simulink model "PFC_Mathematicalmodel_MCHV3"  (R2022a)
settings: Solver=ode8  StartTime=0.0  StopTime=10  RelTol=1e-3
values from neighbouring files (symbols this model uses):
  C = 3*470e-6    (= 0.00141)    [PFC_Mathematicalmodel_MCHV3_data.m]
  Ki_i = Kp_i*2*pi*fz_i    (= 14162.3628627)    [PFC_Mathematicalmodel_MCHV3_data.m]
  Ki_v = Kp_v*2*pi*fz_v    (= 22.7249846961)    [PFC_Mathematicalmodel_MCHV3_data.m]
  KiL = 1/Ibase    (= 0.0469483568075)    [PFC_Mathematicalmodel_MCHV3_data.m]
  Kmul = Vpk_min/(2*Vbase)    (= 0.218498896247)    [PFC_Mathematicalmodel_MCHV3_data.m]
  Kp_i = Gci    (= 2.81751256932)    [PFC_Mathematicalmodel_MCHV3_data.m]
  Kp_v = Gcv    (= 3.61679364607)    [PFC_Mathematicalmodel_MCHV3_data.m]
  Kvin = 1/Vbase    (= 0.00220750551876)    [PFC_Mathematicalmodel_MCHV3_data.m]
  Kvo = 1/Vbase    (= 0.00220750551876)    [PFC_Mathematicalmodel_MCHV3_data.m]
  L = 1e-3    (= 0.001)    [PFC_Mathematicalmodel_MCHV3_data.m]
  R = (Vout^2)/Po    (= 144.4)    [PFC_Mathematicalmodel_MCHV3_data.m]
  Slope = (Vref-Vout_init)/T_rise    (= 273.9)    [PFC_Mathematicalmodel_MCHV3_data.m]
  Tsi = Isr / fsw    (= 1.25e-05)    [PFC_Mathematicalmodel_MCHV3_data.m]
  Tsv = Osr / fsw    (= 0.0002)    [PFC_Mathematicalmodel_MCHV3_data.m]
  Vin_pk = Vin_rms*1.414    (= 325.22)    [PFC_Mathematicalmodel_MCHV3_data.m]
  Vin_rms = 230    [PFC_Mathematicalmodel_MCHV3_data.m]
libraries: slpidlib x2, simulink x2, spsPWMGeneratorDCDCLib x1, spsRMSLib x1, spsMeanLib x1
settings Model: Creator=I50990  LastModifiedBy=I50990

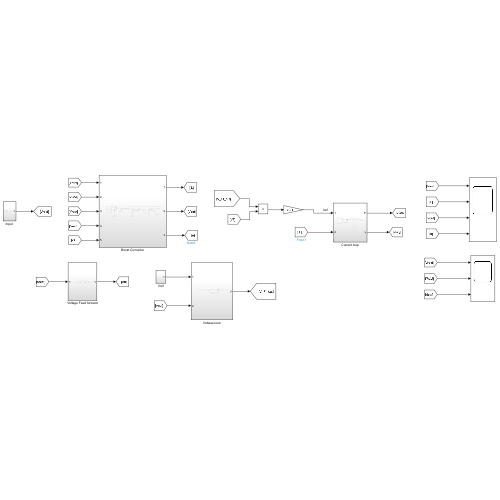
[thumbnail: Simulink's stored preview of the top-level diagram]
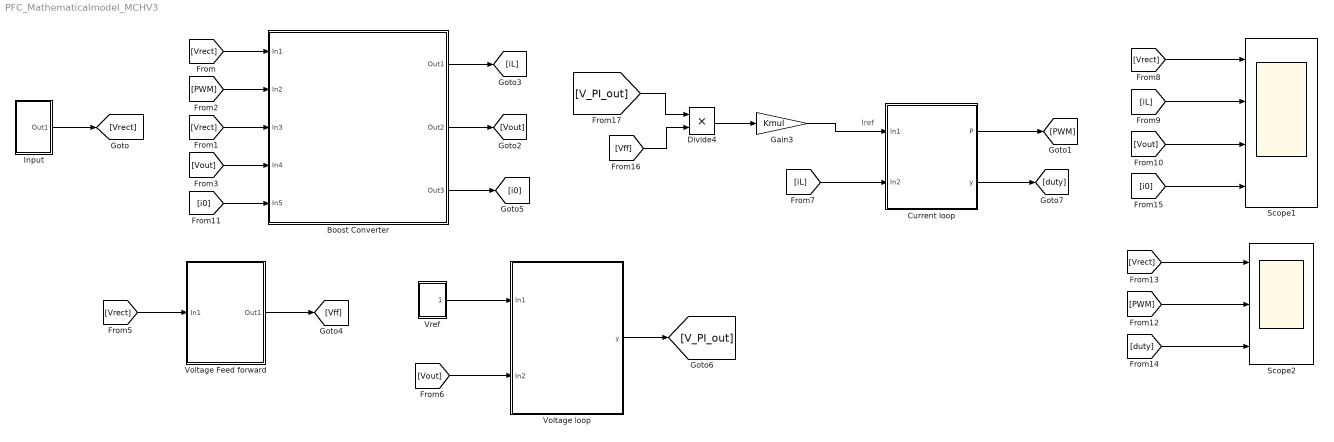
== system PFC_Mathematicalmodel_MCHV3 ==
  note: Iref
  Boost Converter : Subsystem
  Current loop : Subsystem
  Divide4 : Product  Inputs=**
  Gain3 : Gain  Gain=Kmul
  "Input " : Subsystem
  Scope1 : Scope  NumInputPorts=4
  Scope2 : Scope  NumInputPorts=3
  Voltage Feed forward : Subsystem
  Voltage loop : Subsystem
  Vref : Subsystem
  wires:
  Divide4/1 -> Gain3/1
  [Vrect] -> Scope1/1
  [iL] -> Scope1/2
  [Vout] -> Scope1/3
  [duty] -> Scope2/3
  [PWM] -> Scope2/2
  [Vrect] -> Scope2/1
  [i0] -> Scope1/4
  "Input "/1(Out1) -> [Vrect]
  [Vff] -> Divide4/2
  [V_PI_out] -> Divide4/1
  Vref/1(Out1) -> Voltage loop/1(In1)
  [Vout] -> Voltage loop/2(In2)
  Voltage loop/1(y) -> [V_PI_out]
  [Vrect] -> Boost Converter/1(In1)
  [PWM] -> Boost Converter/2(In2)
  [Vrect] -> Boost Converter/3(In3)
  [Vout] -> Boost Converter/4(In4)
  [i0] -> Boost Converter/5(In5)
  Boost Converter/1(Out1) -> [iL]
  Boost Converter/2(Out2) -> [Vout]
  Boost Converter/3(Out3) -> [i0]
  [Vrect] -> Voltage Feed forward/1(In1)
  Voltage Feed forward/1(Out1) -> [Vff]
  Gain3/1 -> Current loop/1(In1)
  [iL] -> Current loop/2(In2)
  Current loop/1(P) -> [PWM]
  Current loop/2(y) -> [duty]

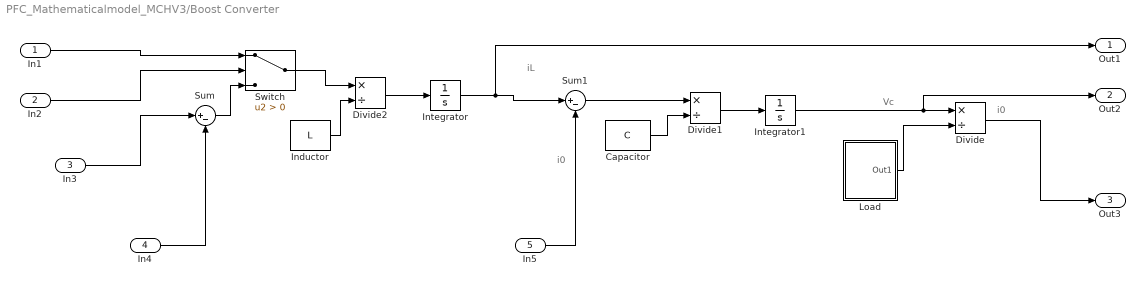
== system PFC_Mathematicalmodel_MCHV3/Boost Converter ==
  note: i0
  note: Vc
  note: i0
  note: iL
  In1 : Inport
  In2 : Inport  Port=2
  In3 : Inport  Port=3
  In4 : Inport  Port=4
  In5 : Inport  Port=5
  Capacitor : Constant  Value=C  SampleTime=Tsi
  Divide : Product  Inputs=*/
  Divide1 : Product  Inputs=*/
  Divide2 : Product  Inputs=*/
  Inductor : Constant  Value=L  SampleTime=Tsi
  Integrator : Integrator
  Integrator1 : Integrator  InitialCondition=Vin_pk
  Load : Subsystem
  Sum : Sum  Inputs=|+-
  Sum1 : Sum  Inputs=|+-
  Switch : Switch  Criteria=u2 > Threshold  SaturateOnIntegerOverflow=off  InputSameDT=off
  Out1 : Outport
  Out2 : Outport  Port=2
  Out3 : Outport  Port=3
  wires:
  Sum/1 -> Switch/3
  Integrator/1 -> Out1/1, Sum1/1
  In3/1 -> Sum/1
  Divide/1 -> Out3/1
  Integrator1/1 -> Out2/1, Divide/1
  Capacitor/1 -> Divide1/2
  In1/1 -> Switch/1
  Load/1(Out1) -> Divide/2
  Divide2/1 -> Integrator/1
  Divide1/1 -> Integrator1/1
  Switch/1 -> Divide2/1
  Sum1/1 -> Divide1/1
  Inductor/1 -> Divide2/2
  In5/1 -> Sum1/2
  In2/1 -> Switch/2
  In4/1 -> Sum/2

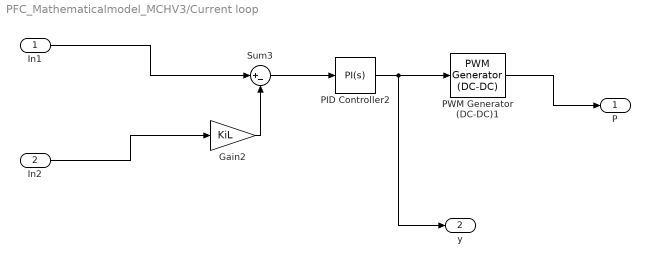
== system PFC_Mathematicalmodel_MCHV3/Current loop ==
  In1 : Inport
  In2 : Inport  Port=2
  Gain2 : Gain  Gain=KiL
  PID Controller2 : slpidlib/PID Controller  Controller=PI  Form=Parallel  TimeDomain=Continuous-time  UseExternalTs=off  SampleTime=-1  IntegratorMethod=Forward Euler  FilterMethod=Forward Euler  ControllerParametersSource=internal  P=Kp_i  I=Ki_i  UseKiTs=off  D=0  N=100  UseFilter=on  TunerSelectOption=Transfer Function Based (PID Tuner App)  ZeroCross=off  InitialConditionSource=internal  InitialConditionForIntegrator=0  InitialConditionForFilter=0  DifferentiatorICPrevScaledInput=0  ExternalReset=none  TrackingMode=off  Kt=1  LimitOutput=on  SatLimitsSource=internal  UpperSaturationLimit=0.95  LowerSaturationLimit=0  LinearizeAsGain=on  AntiWindupMode=none  Kb=1  POutMin=[]  POutMax=[]  IOutMin=[]  IOutMax=[]  DOutMin=[]  DOutMax=[]  NOutMin=[]  NOutMax=[]  SumOutMin=[]  SumOutMax=[]  SaturationOutMin=[]  SaturationOutMax=[]  PParamMin=[]  PParamMax=[]  IParamMin=[]  IParamMax=[]  DParamMin=[]  DParamMax=[]  NParamMin=[]  NParamMax=[]  KbParamMin=[]  KbParamMax=[]  KtParamMin=[]  KtParamMax=[]  KbOutMin=[]  KbOutMax=[]  KtOutMin=[]  KtOutMax=[]  IntegratorOutMin=[]  IntegratorOutMax=[]  FilterOutMin=[]  FilterOutMax=[]  SumI1OutMin=[]  SumI1OutMax=[]  SumI2OutMin=[]  SumI2OutMax=[]  SumI3OutMin=[]  SumI3OutMax=[]  SumI4OutMin=[]  SumI4OutMax=[]  SumDOutMin=[]  SumDOutMax=[]  DifferentiatorOutMin=[]  DifferentiatorOutMax=[]  FilterDiffOutCoefMin=[]  FilterDiffOutCoefMax=[]  ReciprocalOutMin=[]  ReciprocalOutMax=[]  SumDenOutMin=[]  SumDenOutMax=[]  SumNumOutMin=[]  SumNumOutMax=[]  DivideOutMin=[]  DivideOutMax=[]  UdiffTsProdOutMin=[]  UdiffTsProdOutMax=[]  NTsProdOutMin=[]  NTsProdOutMax=[]  UintegralTsProdOutMin=[]  UintegralTsProdOutMax=[]  UngainTsProdOutMin=[]  UngainTsProdOutMax=[]  IntegratorContinuousStateAttributes=''  IntegratorStateMustResolveToSignalObject=off  IntegratorRTWStateStorageClass=Auto  FilterContinuousStateAttributes=''  FilterStateMustResolveToSignalObject=off  FilterRTWStateStorageClass=Auto  ParallelPVariant=InternalParameters  IdealPVariant=Disabled  IVariant=InternalParameters  DVariant=Disabled  IntegratorVariant=Continuous  SatVariant=Enabled  AWVariant=Passthrough  PCopyVariant=Disabled  TRVariant=Disabled  FdbkBlocksVariant=Forward  IdealPFdbkVariant=Disabled  SatFdbkVariant=Disabled  DerivativeFilterVariant=Disabled  NVariant=Disabled  NCopyVariant=Disabled_SignalSpec  FilterICVariant=Disabled  IntegratorICVariant=InternalICs  ExternalResetVariant=Disabled  TRSumVariant=Passthrough  SumFdbkVariant=Disabled  SumVariant=Sum_PI  TsampFilterVariant=InternalTs  TsampNgainVariant=Passthrough  TsampIntegralVariant=Passthrough  ExternalSaturationOutDataTypeStr=Inherit: Same as second input  aMode=0
  PWM Generator (DC-DC)1 : spsPWMGeneratorDCDCLib/PWM Generator (DC-DC)  Fsw=fsw  Ts=Tsi/10
  Sum3 : Sum  Inputs=|+-
  P : Outport
  y : Outport  Port=2
  wires:
  Gain2/1 -> Sum3/2
  In2/1 -> Gain2/1
  Sum3/1 -> PID Controller2/1
  In1/1 -> Sum3/1
  PID Controller2/1 -> y/1, PWM Generator (DC-DC)1/1
  PWM Generator (DC-DC)1/1 -> P/1

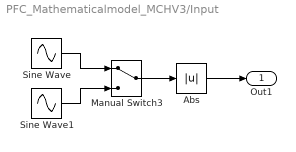
== system PFC_Mathematicalmodel_MCHV3/Input  ==
  Abs : Abs  SaturateOnIntegerOverflow=off
  Manual Switch3 : ManualSwitch
  Sine Wave : Sin  Amplitude=Vin_pk  Frequency=2*pi*50  SampleTime=0
  Sine Wave1 : Sin  Amplitude=Vin_pk/2  Frequency=2*pi*50  SampleTime=0
  Out1 : Outport
  wires:
  Sine Wave/1 -> Manual Switch3/1
  Manual Switch3/1 -> Abs/1
  Sine Wave1/1 -> Manual Switch3/2
  Abs/1 -> Out1/1

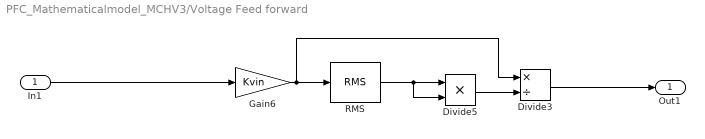
== system PFC_Mathematicalmodel_MCHV3/Voltage Feed forward ==
  In1 : Inport
  Divide3 : Product  Inputs=*/
  Divide5 : Product  Inputs=**
  Gain6 : Gain  Gain=Kvin
  RMS : spsRMSLib/RMS  TrueRMS=on  Freq=100  RMSInit=Vin_rms*Kvin  Ts=Tsi
  Out1 : Outport
  wires:
  RMS/1 -> Divide5/2, Divide5/1
  Gain6/1 -> Divide3/1, RMS/1
  Divide3/1 -> Out1/1
  Divide5/1 -> Divide3/2
  In1/1 -> Gain6/1

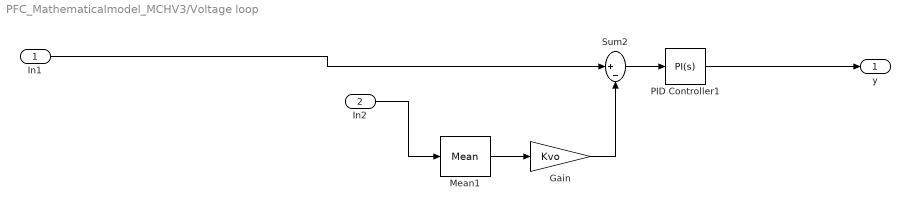
== system PFC_Mathematicalmodel_MCHV3/Voltage loop ==
  In1 : Inport
  In2 : Inport  Port=2
  Gain : Gain  Gain=Kvo
  Mean1 : spsMeanLib/Mean  Freq=100  Vinit=Vin_pk  Ts=Tsv
  PID Controller1 : slpidlib/PID Controller  Controller=PI  Form=Parallel  TimeDomain=Continuous-time  UseExternalTs=off  SampleTime=-1  IntegratorMethod=Forward Euler  FilterMethod=Forward Euler  ControllerParametersSource=internal  P=Kp_v  I=Ki_v  UseKiTs=off  D=0  N=100  UseFilter=on  TunerSelectOption=Transfer Function Based (PID Tuner App)  InitialConditionSource=internal  InitialConditionForIntegrator=0  InitialConditionForFilter=0  DifferentiatorICPrevScaledInput=0  ExternalReset=none  TrackingMode=off  Kt=1  LimitOutput=on  SatLimitsSource=internal  UpperSaturationLimit=1  LowerSaturationLimit=0  LinearizeAsGain=on  AntiWindupMode=none  Kb=1  POutMin=[]  POutMax=[]  IOutMin=[]  IOutMax=[]  DOutMin=[]  DOutMax=[]  NOutMin=[]  NOutMax=[]  SumOutMin=[]  SumOutMax=[]  SaturationOutMin=[]  SaturationOutMax=[]  PParamMin=[]  PParamMax=[]  IParamMin=[]  IParamMax=[]  DParamMin=[]  DParamMax=[]  NParamMin=[]  NParamMax=[]  KbParamMin=[]  KbParamMax=[]  KtParamMin=[]  KtParamMax=[]  KbOutMin=[]  KbOutMax=[]  KtOutMin=[]  KtOutMax=[]  IntegratorOutMin=[]  IntegratorOutMax=[]  FilterOutMin=[]  FilterOutMax=[]  SumI1OutMin=[]  SumI1OutMax=[]  SumI2OutMin=[]  SumI2OutMax=[]  SumI3OutMin=[]  SumI3OutMax=[]  SumI4OutMin=[]  SumI4OutMax=[]  SumDOutMin=[]  SumDOutMax=[]  DifferentiatorOutMin=[]  DifferentiatorOutMax=[]  FilterDiffOutCoefMin=[]  FilterDiffOutCoefMax=[]  ReciprocalOutMin=[]  ReciprocalOutMax=[]  SumDenOutMin=[]  SumDenOutMax=[]  SumNumOutMin=[]  SumNumOutMax=[]  DivideOutMin=[]  DivideOutMax=[]  UdiffTsProdOutMin=[]  UdiffTsProdOutMax=[]  NTsProdOutMin=[]  NTsProdOutMax=[]  UintegralTsProdOutMin=[]  UintegralTsProdOutMax=[]  UngainTsProdOutMin=[]  UngainTsProdOutMax=[]  IntegratorContinuousStateAttributes=''  IntegratorStateMustResolveToSignalObject=off  IntegratorRTWStateStorageClass=Auto  FilterContinuousStateAttributes=''  FilterStateMustResolveToSignalObject=off  FilterRTWStateStorageClass=Auto  ParallelPVariant=InternalParameters  IdealPVariant=Disabled  IVariant=InternalParameters  DVariant=Disabled  IntegratorVariant=Continuous  SatVariant=Enabled  AWVariant=Passthrough  PCopyVariant=Disabled  TRVariant=Disabled  FdbkBlocksVariant=Forward  IdealPFdbkVariant=Disabled  SatFdbkVariant=Disabled  DerivativeFilterVariant=Disabled  NVariant=Disabled  NCopyVariant=Disabled_SignalSpec  FilterICVariant=Disabled  IntegratorICVariant=InternalICs  ExternalResetVariant=Disabled  TRSumVariant=Passthrough  SumFdbkVariant=Disabled  SumVariant=Sum_PI  TsampFilterVariant=InternalTs  TsampNgainVariant=Passthrough  TsampIntegralVariant=Passthrough  ExternalSaturationOutDataTypeStr=Inherit: Same as second input  aMode=0
  Sum2 : Sum  Inputs=|+-
  y : Outport
  wires:
  In2/1 -> Mean1/1
  Sum2/1 -> PID Controller1/1
  Mean1/1 -> Gain/1
  In1/1 -> Sum2/1
  Gain/1 -> Sum2/2
  PID Controller1/1 -> y/1

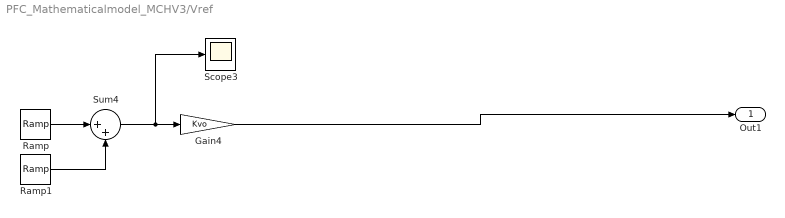
== system PFC_Mathematicalmodel_MCHV3/Vref ==
  Gain4 : Gain  Gain=Kvo
  Ramp : simulink/Sources/Ramp  slope=Slope  start=0  InitialOutput=Vin_pk
  Ramp1 : simulink/Sources/Ramp  slope=-Slope  start=T_rise  InitialOutput=0
  Scope3 : Scope
  Sum4 : Sum  Inputs=|++
  Out1 : Outport
  wires:
  Gain4/1 -> Out1/1
  Ramp1/1 -> Sum4/2
  Ramp/1 -> Sum4/1
  Sum4/1 -> Scope3/1, Gain4/1

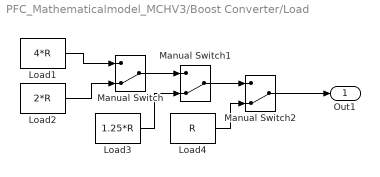
== system PFC_Mathematicalmodel_MCHV3/Boost Converter/Load ==
  Load1 : Constant  Value=4*R  SampleTime=Tsi
  Load2 : Constant  Value=2*R  SampleTime=Tsi
  Load3 : Constant  Value=1.25*R  SampleTime=Tsi
  Load4 : Constant  Value=R  SampleTime=Tsi
  Manual Switch : ManualSwitch  CurrentSetting=0
  Manual Switch1 : ManualSwitch  CurrentSetting=0
  Manual Switch2 : ManualSwitch  CurrentSetting=0
  Out1 : Outport
  wires:
  Load3/1 -> Manual Switch1/2
  Load2/1 -> Manual Switch/2
  Manual Switch1/1 -> Manual Switch2/1
  Load4/1 -> Manual Switch2/2
  Manual Switch2/1 -> Out1/1
  Manual Switch/1 -> Manual Switch1/1
  Load1/1 -> Manual Switch/1
